simulink model "edgeDet_try2"  (R2013b)
settings: Solver=ode45  StartTime=0.0  StopTime=10.0  RelTol=1e-3
settings Model: Creator=aidan  LastModifiedBy=aidan

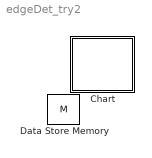
== system edgeDet_try2 ==
  Chart : Stateflow chart  TreatAsAtomicUnit=on
  Data Store Memory : DataStoreMemory  DataStoreName=M  ReadBeforeWriteMsg=warning  WriteAfterWriteMsg=warning  WriteAfterReadMsg=warning  Dimensions=20:20

== stateflow chart edgeDet_try2/Chart ==
  state Convert Image to GrayScale [group]
    state ?
  state Calculate Intensity Stuff [group]
    state Write to File
      #Write to the Really big Matrix
    state Increment
      x=x+1;
      #If x mod something == 0
      y=y+1;
    state x=1;
      y=1;
    state Do_Math
      Gx = [-1 0 1; -2 0 2;-1 0 1];
      Gy = [1 2 1;  0 0 0; -1 -2 -1];
      SUM_X = 0;
      SUM_Y = 0;
      for i = 1:3
      for j = 1:3
      if(i != 2, j != 2)
      SUM_X = SUM_X + Gx(i, j) * A(i,j);
      SUM_Y = SUM_Y + Gy(i, j) * A(i,j);
      end
      end
      end
    state Select_Matrix
      A = M[1](x-1:x+1,y-1:y+1);
    Write to File -> Increment : 1
    x=1; -> Select_Matrix
    Increment -> Select_Matrix : 1
    Do_Math -> Write to File : 1
    Select_Matrix -> Do_Math [order 1] : if NOT if x,y == (width-1,height-1)
  state Split Image Up [group]
    state NothingForNow
      #Just pass same image through
  (default) -> x=1;
  Select_Matrix -> (junction 27) [order 2] : if x,y == (width-1,height-1)
  data: x local double; y local double; M data_store_memory
